simulink model "MBK_DDPG_I"  (R2024a)
settings: Solver=ode45  StartTime=0.0  StopTime=Tf  RelTol=1e-5  AbsTol=1e-6
model workspace (MAT data in the model file):
  I = 0
  c = 0
  g = 9.81
  l = 1
  m = 1
  max_tau = 2
  theta0 = 0
  theta_dot0 = 0
values from neighbouring files (symbols this model uses):
  b = 2    [CreateSimulinkEnvironmentTrainAgentMBK.m]    (also in CreateSimulinkEnvironmentTrainAgentMBK_I.m)
  k = 5    [CreateSimulinkEnvironmentTrainAgentMBK.m]    (also in CreateSimulinkEnvironmentTrainAgentMBK_I.m)
undefined symbols (not defined in the file or in its folder): x0
libraries: rllib x1
settings Model: Creator=The MathWorks, Inc.  LastModifiedBy=Ali
settings SolverCC: AutoScaleAbsTol=off  AlgebraicLoopSolver=TrustRegion
settings DataIOCC: LimitDataPoints=on  SaveFormat=Array  SaveState=on
settings OptimizationCC: BlockReduction=off  BooleanDataType=off  LifeSpan=inf
settings DebuggingCC: SaveWithParameterizedLinksMsg=none  SignalResolutionControl=TryResolveAllWithWarning  UnconnectedInputMsg=warning  UnconnectedOutputMsg=warning  UnconnectedLineMsg=warning  SFUnexpectedBacktrackingDiag=warning  SFNoUnconditionalDefaultTransitionDiag=warning  SFExecutionAtInitializationDiag=none  ArithmeticOperatorsInVariantConditions=warning
settings HardwareCC: ProdBitPerPointer=32  ProdBitPerSizeT=32  ProdBitPerPtrDiffT=32  ProdLargestAtomicFloat=None  ProdIntDivRoundTo=Undefined  ProdEndianess=Unspecified  ProdWordSize=32  ProdHWDeviceType=32-bit Generic  TargetUnknown=on
settings ModelReferenceCC: EnableRefExpFcnMdlSchedulingChecks=on  PropagateSignalLabelsOutOfModel=off
settings SFSimCC: SimUseLocalCustomCode=off  CustomCodeUndefinedFunction=UseInterfaceOnly
settings RTWCC: RTWUseLocalCustomCode=off  GPUComputeCapability=3.5
settings CodeAppCC: StateflowObjectComments=on
settings GRTTargetCC: TargetLangStandard=C89/C90 (ANSI)
settings ConfigComp: CovMetricSettings=dw  CovSaveCumulativeToWorkspaceVar=on  CovSaveSingleToWorkspaceVar=on  CovExternalEMLEnable=off

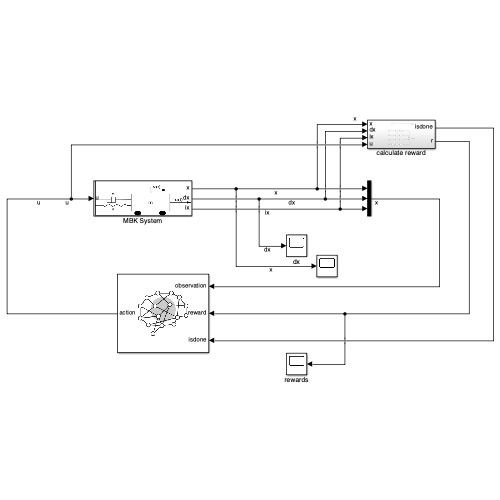
[thumbnail: Simulink's stored preview of the top-level diagram]
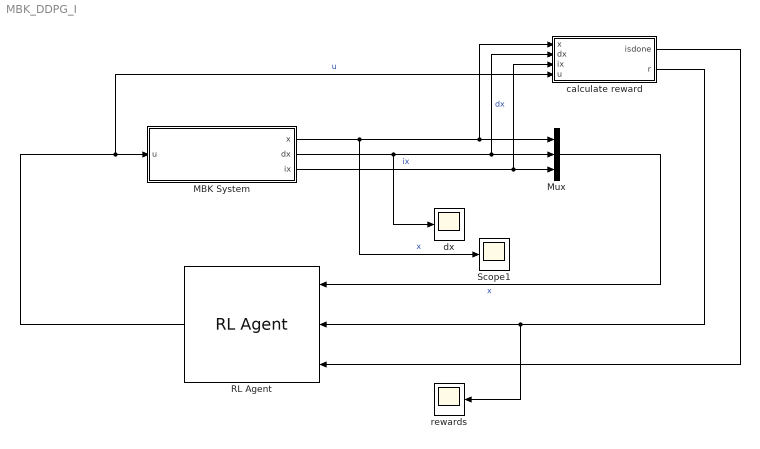
== system MBK_DDPG_I ==
  MBK System : Subsystem
      mask Display: image('MBKPic.png');
  Mux : Mux  Inputs=3
  RL Agent : rllib/RL Agent  Agent=agent  ExternalActionAsInput=off  ProvideLastAction=off  ProvideCumRwd=off  TreatAsDirectFeedthrough=on  UseStrictObservationDataTypes=off
  Scope1 : Scope
  calculate reward : Subsystem
  dx : Scope
  rewards : Scope
  wires:
  MBK System/2(dx) -> dx/1, calculate reward/2(dx), Mux/2  "dx"
  MBK System/1(x) -> calculate reward/1(x), Mux/1, Scope1/1  "x"
  calculate reward/2(r) -> rewards/1, RL Agent/2
  calculate reward/1(isdone) -> RL Agent/3
  RL Agent/1 -> MBK System/1(u), calculate reward/4(u)  "u"
  Mux/1 -> RL Agent/1  "x"
  MBK System/3(ix) -> calculate reward/3(ix), Mux/3  "ix"

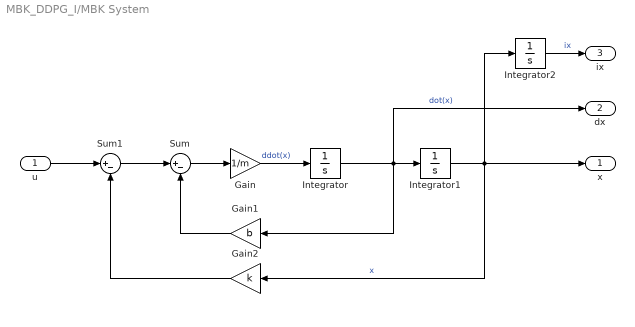
== system MBK_DDPG_I/MBK System ==
  u : Inport
  Gain : Gain  Gain=1/m
  Gain1 : Gain  Gain=b
  Gain2 : Gain  Gain=k
  Integrator : Integrator
  Integrator1 : Integrator  InitialCondition=x0
  Integrator2 : Integrator
  Sum : Sum  Inputs=|+-
  Sum1 : Sum  Inputs=|+-
  x : Outport
  dx : Outport  Port=2
  ix : Outport  Port=3
  wires:
  Gain2/1 -> Sum1/2
  Gain/1 -> Integrator/1  "ddot(x)"
  Integrator/1 -> dx/1, Gain1/1, Integrator1/1  "dot(x)"
  u/1 -> Sum1/1
  Sum/1 -> Gain/1
  Gain1/1 -> Sum/2
  Integrator1/1 -> Integrator2/1, x/1, Gain2/1  "x"
  Sum1/1 -> Sum/1
  Integrator2/1 -> ix/1  "ix"

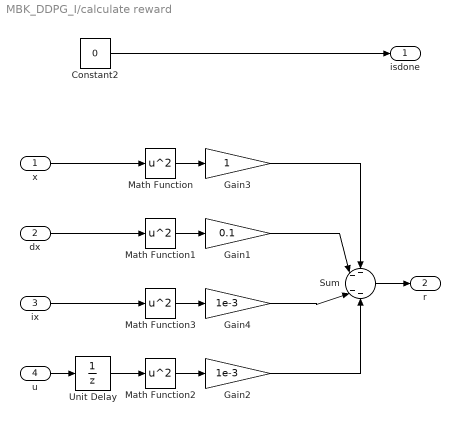
== system MBK_DDPG_I/calculate reward ==
  x : Inport
  dx : Inport  Port=2
  ix : Inport  Port=3
  u : Inport  Port=4
  Constant2 : Constant  Value=0
  Gain1 : Gain  Gain=0.1
  Gain2 : Gain  Gain=1e-3
  Gain3 : Gain
  Gain4 : Gain  Gain=1e-3
  Math Function{,1..3} (4 alike) : Math  Operator=square  SignedPower=on
  Sum : Sum  Inputs=--|--
  Unit Delay : UnitDelay  SampleTime=-1  HasFrameUpgradeWarning=on
  isdone : Outport  VectorParamsAs1DForOutWhenUnconnected=off
  r : Outport  Port=2  VectorParamsAs1DForOutWhenUnconnected=off
  wires:
  Constant2/1 -> isdone/1
  x/1 -> Math Function/1
  dx/1 -> Math Function1/1
  u/1 -> Unit Delay/1
  Sum/1 -> r/1
  Math Function/1 -> Gain3/1
  Math Function1/1 -> Gain1/1
  Math Function2/1 -> Gain2/1
  Gain1/1 -> Sum/2
  Gain3/1 -> Sum/1
  Unit Delay/1 -> Math Function2/1
  Math Function3/1 -> Gain4/1
  ix/1 -> Math Function3/1
  Gain2/1 -> Sum/4
  Gain4/1 -> Sum/3
